simulink model "simulation"  (R2019b)
settings: Solver=VariableStepAuto  StartTime=0.0  StopTime=25.0  RelTol=1e-3
values from neighbouring files (symbols this model uses):
  beta = [b_gb_lw; b_gb_rw; b_t]    [config.m]
  g = 9.8    [config.m]
  J = [Jbphi; Jbpsi; Jm; Jw]    [config.m]
  K_enc = 1    [config.m]
  K_gyro = 1    [config.m]
  M = [Mb; Mw]    [config.m]
  params = [L; W; R; eta]    [config.m]
  Q = 10    [NMPC_controller.m]    (also in config.m = eta*K_mot*K_da*[K_amp_lw, 0; 0, K_amp_rw; -K_amp_lw, -K_amp_)
  q_dot_inital = [0; 0; 0]    [config.m]
  q_inital = [0; 0; 0]    [config.m]
undefined symbols (not defined in the file or in its folder): q_dot_initial, q_initial, sigbuilder_block, x_initial, y_initial
libraries: simulink x1
settings Model: Creator=nishantmittal  LastModifiedBy=nishantmittal

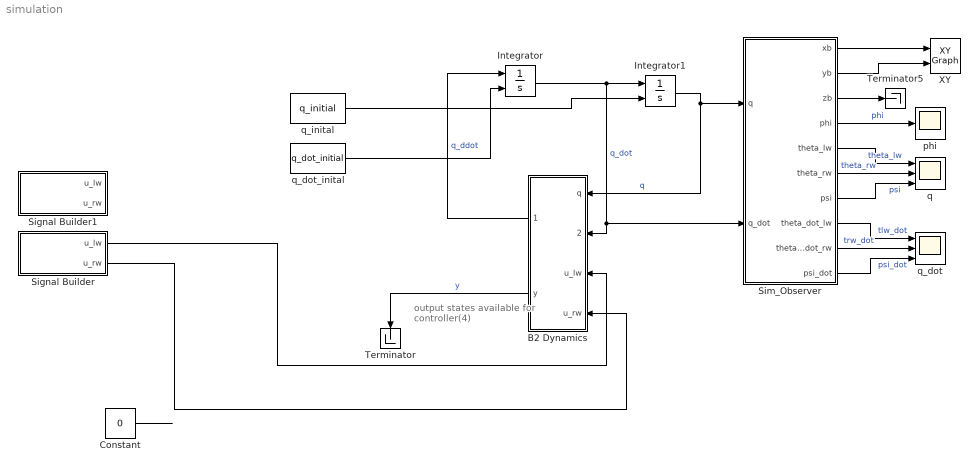
== system simulation ==
  note: output states available
      | for controller(4)
  "B2 Dynamics " : Subsystem
  Constant : Constant  Value=0
  Integrator : Integrator  InitialConditionSource=external  InitialCondition=q_dot_inital
  Integrator1 : Integrator  InitialConditionSource=external  InitialCondition=q_inital
  Signal Builder : Subsystem  Tag=STV Subsys  LoadFcn=sigbuilder_block('load');  StartFcn=sigbuilder_block('start');  StopFcn=sigbuilder_block('stop');  ClipboardFcn=sigbuilder_block('clipboard');  mask(Sigbuilder block){tuvar=[0:10]}
      mask help: Simulink:masks:SigbuilderBlock_MD
      mask init:
      | if ~strcmp(get_param(bdroot(gcbh),'SimulationStatus'),'stopped') tuvar = sigbuilder_block('maskInit'); end
      settings: CopyFcn=sigbuilder_block('copy');  DeleteFcn=sigbuilder_block('delete');  ModelCloseFcn=sigbuilder_block('modelClose');  PreSaveFcn=sigbuilder_block('preSave');  PauseFcn=sigbuilder_block('pause');  ContinueFcn=sigbuilder_block('continue');  NameChangeFcn=sigbuilder_block('namechange');  OpenFcn=sigbuilder_block('open',[436 201 612 537 ]);  CloseFcn=sigbuilder_block('close');
      mask Display: plot(0, 0, 100, 100,[2, 2, 32, 32, 2], [68, 8, 8, 68, 68],[32, 2], [38, 38], [32, 19, 2],[53, 60, 44], [32, 17, 17, 2],[16, 16, 31, 31]);txt = getActiveGroup(gcbh);text(2, 100, txt,'verticalAlignment', 'top');
  Signal Builder1 : Subsystem  Tag=STV Subsys  LoadFcn=sigbuilder_block('load');  StartFcn=sigbuilder_block('start');  StopFcn=sigbuilder_block('stop');  ClipboardFcn=sigbuilder_block('clipboard');  mask(Sigbuilder block){tuvar=[0:10]}
      mask help: Simulink:masks:SigbuilderBlock_MD
      mask init:
      | if ~strcmp(get_param(bdroot(gcbh),'SimulationStatus'),'stopped') tuvar = sigbuilder_block('maskInit'); end
      settings: CopyFcn=sigbuilder_block('copy');  DeleteFcn=sigbuilder_block('delete');  ModelCloseFcn=sigbuilder_block('modelClose');  PreSaveFcn=sigbuilder_block('preSave');  PauseFcn=sigbuilder_block('pause');  ContinueFcn=sigbuilder_block('continue');  NameChangeFcn=sigbuilder_block('namechange');  OpenFcn=sigbuilder_block('open',[436 201 612 537 ]);  CloseFcn=sigbuilder_block('close');
      mask Display: plot(0, 0, 100, 100,[2, 2, 32, 32, 2], [68, 8, 8, 68, 68],[32, 2], [38, 38], [32, 19, 2],[53, 60, 44], [32, 17, 17, 2],[16, 16, 31, 31]);txt = getActiveGroup(gcbh);text(2, 100, txt,'verticalAlignment', 'top');
  Sim_Observer : Subsystem
  Terminator : Terminator
  Terminator5 : Terminator
  XY : simulink/Sinks/XY Graph  xmin=-25  xmax=25  ymin=-25  ymax=25  st=-1
  phi : Scope
  q : Scope  NumInputPorts=3
  q_dot : Scope  NumInputPorts=3
  q_dot_inital : Constant  Value=q_dot_initial
  q_inital : Constant  Value=q_initial
  wires:
  Integrator/1 -> "B2 Dynamics "/2(q_dot), Sim_Observer/2(q_dot), Integrator1/1  "q_dot"
  Integrator1/1 -> Sim_Observer/1(q), "B2 Dynamics "/1(q)  "q"
  "B2 Dynamics "/1(q_ddot) -> Integrator/1  "q_ddot"
  "B2 Dynamics "/2(y) -> Terminator/1  "y"
  q_dot_inital/1 -> Integrator/2
  q_inital/1 -> Integrator1/2
  Sim_Observer/6(theta_rw) -> q/2  "theta_rw"
  Sim_Observer/5(theta_lw) -> q/1  "theta_lw"
  Sim_Observer/7(psi) -> q/3  "psi"
  Sim_Observer/2(yb) -> XY/2
  Sim_Observer/1(xb) -> XY/1
  Sim_Observer/10(psi_dot) -> q_dot/3  "psi_dot"
  Sim_Observer/9(theta_dot_rw) -> q_dot/2  "trw_dot"
  Sim_Observer/8(theta_dot_lw) -> q_dot/1  "tlw_dot"
  Sim_Observer/4("phi ") -> phi/1  "phi"
  Sim_Observer/3(zb) -> Terminator5/1
  Constant/1 -> ?
  Signal Builder/1(u_lw) -> "B2 Dynamics "/3(u_lw)
  Signal Builder/2(u_rw) -> "B2 Dynamics "/4(u_rw)

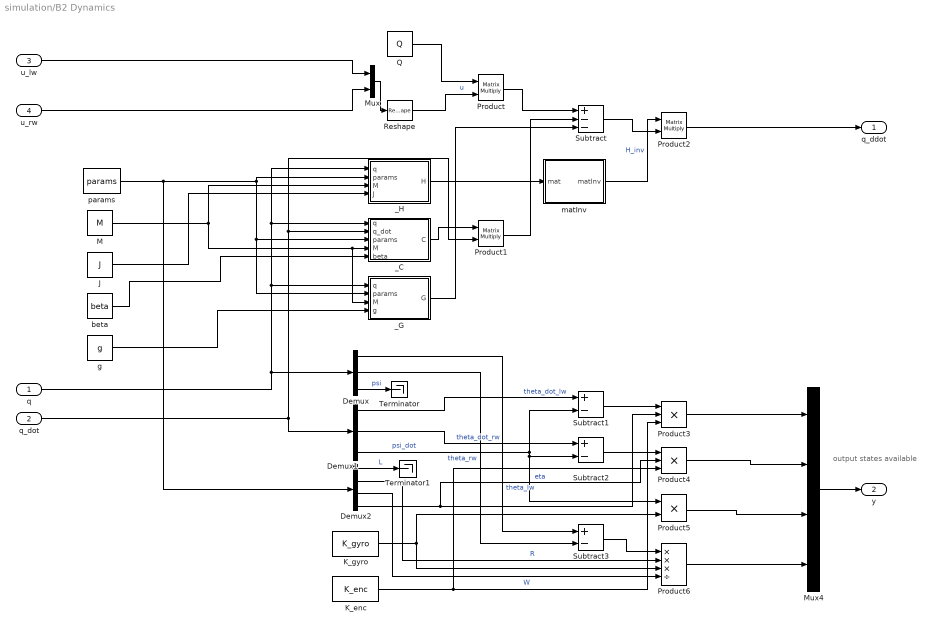
== system simulation/B2 Dynamics  ==
  note: output states available
  q : Inport
  q_dot : Inport  Port=2
  u_lw : Inport  Port=3
  u_rw : Inport  Port=4
  Demux : Demux  Outputs=3
  Demux1 : Demux  Outputs=3
  Demux2 : Demux
  J : Constant  Value=J
  K_enc : Constant  Value=K_enc
  K_gyro : Constant  Value=K_gyro
  M : Constant  Value=M
  Mux : Mux  Inputs=2
  Mux4 : Mux
  Product : Product  Multiplication=Matrix(*)
  Product1 : Product  Multiplication=Matrix(*)
  Product2 : Product  Multiplication=Matrix(*)
  Product3 : Product  Inputs=3
  Product4 : Product  Inputs=3
  Product5 : Product
  Product6 : Product  Inputs=***/
  Q : Constant  Value=Q
  Reshape : Reshape  OutputDimensionality=Column vector (2-D)
  Subtract : Sum  Inputs=+--
  Subtract1 : Sum  Inputs=+-
  Subtract2 : Sum  Inputs=+-
  Subtract3 : Sum  Inputs=+-
  Terminator : Terminator
  Terminator1 : Terminator
  _C : MATLAB Function  TreatAsAtomicUnit=on
  _G : MATLAB Function  TreatAsAtomicUnit=on
  _H : MATLAB Function  TreatAsAtomicUnit=on
  beta : Constant  Value=beta
  g : Constant  Value=g
  matInv : MATLAB Function  TreatAsAtomicUnit=on
  "params " : Constant  Value=params
  q_ddot : Outport
  y : Outport  Port=2
  wires:
  q_dot/1 -> _C/2(q_dot), Product1/2, Demux1/1
  "params "/1 -> Demux2/1, _G/2(params), _C/3(params), _H/2(params)
  beta/1 -> _C/5(beta)
  J/1 -> _H/4(J)
  M/1 -> _H/3(M), _G/3(M), _C/4(M)
  g/1 -> _G/4(g)
  u_rw/1 -> Mux/2
  u_lw/1 -> Mux/1
  Mux/1 -> Reshape/1
  _H/1(H) -> matInv/1(mat)
  Product/1 -> Subtract/1
  Product1/1 -> Subtract/2
  _G/1(G) -> Subtract/3
  Product2/1 -> q_ddot/1
  Demux/1 -> Subtract3/1  "theta_lw"
  Demux/2 -> Subtract3/2  "theta_rw"
  Demux1/1 -> Subtract1/1  "theta_dot_lw"
  Subtract1/1 -> Product3/1
  Demux2/2 -> Product6/2  "R"
  Demux2/3 -> Product6/4  "W"
  K_enc/1 -> Product4/3, Product3/3
  Demux1/2 -> Subtract2/1  "theta_dot_rw"
  Subtract2/1 -> Product4/1
  Demux2/4 -> Product4/2, Product3/2  "eta"
  Demux1/3 -> Subtract1/2, Product5/1, Subtract2/2  "psi_dot"
  K_gyro/1 -> Product5/2, Product6/3
  Subtract3/1 -> Product6/1
  Product3/1 -> Mux4/1
  Product4/1 -> Mux4/2
  Product5/1 -> Mux4/3
  Product6/1 -> Mux4/4
  Mux4/1 -> y/1
  Reshape/1 -> Product/2  "u"
  Q/1 -> Product/1
  Subtract/1 -> Product2/2
  matInv/1(matInv) -> Product2/1  "H_inv"
  _C/1(C) -> Product1/1
  Demux/3 -> Terminator/1  "psi"
  Demux2/1 -> Terminator1/1  "L"
  q/1 -> _H/1(q), _C/1(q), _G/1(q), Demux/1

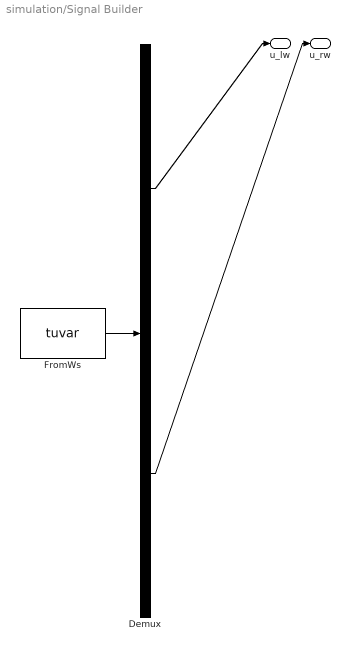
== system simulation/Signal Builder ==
  Demux : Demux  Tag=STV Demux  Outputs=2
  FromWs : FromWorkspace  Tag=STV FromWs  VariableName=tuvar  SampleTime=0
      SigBuilderData=|
      | common.afterFinalStr = 'Extrapolate'
      | common.sampleTime = 0
      | dataSet.timeRange = [0 10]
      | dataSet.name = 'Rotaate'
      | sbobj.Groups.Name = 'Rotaate'
      | sbobj.Groups.Signals(1).Name = 'u_lw'
      | sbobj.Groups.Signals(1).XData = [0 1 1 2 2 3 3 10]
      | sbobj.Groups.Signals(1).YData = [0 0 1.56 1.56 -1.54 -1.54 0 0]
      | sbobj.Groups.Signals(2).Name = 'u_rw'
      | sbobj.Groups.Signals(2).XData = [0 1 1 2 2 3 3 10]
      | sbobj.Groups.Signals(2).YData = [0 0 -1.56 -1.56 1.56 1.56 0 0]
  u_lw : Outport  Tag=STV Outport
  u_rw : Outport  Tag=STV Outport  Port=2
  wires:
  FromWs/1 -> Demux/1
  Demux/1 -> u_lw/1
  Demux/2 -> u_rw/1

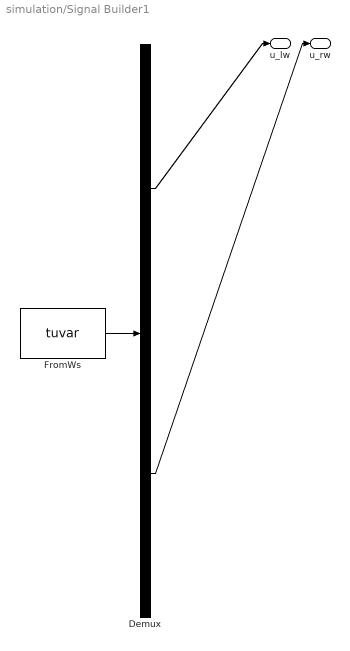
== system simulation/Signal Builder1 ==
  Demux : Demux  Tag=STV Demux  Outputs=2
  FromWs : FromWorkspace  Tag=STV FromWs  VariableName=tuvar  SampleTime=0
      SigBuilderData=|
      | common.afterFinalStr = 'Extrapolate'
      | common.sampleTime = 0
      | dataSet(1).timeRange = [0 10]
      | dataSet(1).name = 'Forward_back'
      | dataSet(2).timeRange = [0 10]
      | dataSet(2).name = 'Group 2'
      | sbobj.Groups(1).Name = 'Forward_back'
      | sbobj.Groups(1).Signals(1).Name = 'u_lw'
      | sbobj.Groups(1).Signals(1).XData = [0 1 1 2 2 3 3 10]
      | sbobj.Groups(1).Signals(1).YData = [0 0 1.56 1.56 -1.54 -1.54 0 0]
      | sbobj.Groups(1).Signals(2).Name = 'u_rw'
      | sbobj.Groups(1).Signals(2).XData = [0 1 1 2 2 3 3 10]
      | sbobj.Groups(1).Signals(2).YData = [0 0 1.56 1.56 -1.56 -1.56 0 0]
      | sbobj.Groups(2).Name = 'Group 2'
      | sbobj.Groups(2).Signals(1).Name = 'u_lw'
      | sbobj.Groups(2).Signals(1).XData = [0 1 1 2 2 3 3 10]
      | sbobj.Groups(2).Signals(1).YData = [0 0 1 1 -1 -1 0 0]
      | sbobj.Groups(2).Signals(2).Name = 'u_rw'
      | sbobj.Groups(2).Signals(2).XData = [0 1 1 2 2 3 3 10]
      | sbobj.Groups(2).Signals(2).YData = [0 0 1 1 -1 -1 0 0]
  u_lw : Outport  Tag=STV Outport
  u_rw : Outport  Tag=STV Outport  Port=2
  wires:
  FromWs/1 -> Demux/1
  Demux/1 -> u_lw/1
  Demux/2 -> u_rw/1

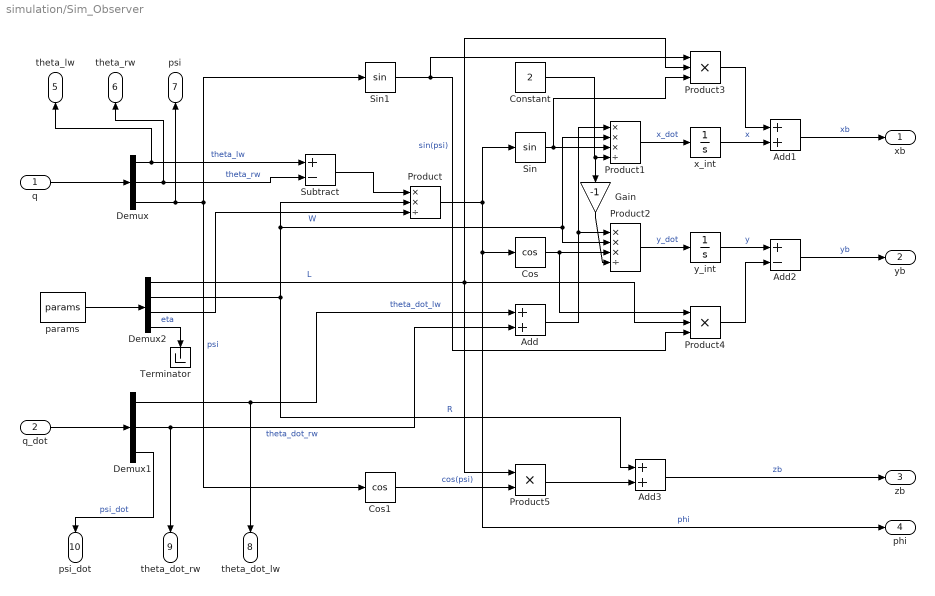
== system simulation/Sim_Observer ==
  q : Inport
  q_dot : Inport  Port=2
  Add : Sum
  Add1 : Sum
  Add2 : Sum  Inputs=+-
  Add3 : Sum
  Constant : Constant  Value=2
  Cos : Trigonometry  Operator=cos
  Cos1 : Trigonometry  Operator=cos
  Demux : Demux  Outputs=3
  Demux1 : Demux  Outputs=3
  Demux2 : Demux
  Gain : Gain  Gain=-1
  Product : Product  Inputs=**/
  Product1 : Product  Inputs=***/
  Product2 : Product  Inputs=***/
  Product3 : Product  Inputs=3
  Product4 : Product  Inputs=3
  Product5 : Product
  Sin : Trigonometry
  Sin1 : Trigonometry
  Subtract : Sum  Inputs=+-
  Terminator : Terminator
  "params " : Constant  Value=params
  x_int : Integrator  InitialCondition=x_initial
  y_int : Integrator  InitialCondition=y_initial
  xb : Outport
  yb : Outport  Port=2
  zb : Outport  Port=3
  "phi " : Outport  Port=4
  theta_lw : Outport  Port=5
  theta_rw : Outport  Port=6
  psi : Outport  Port=7
  theta_dot_lw : Outport  Port=8
  theta_dot_rw : Outport  Port=9
  psi_dot : Outport  Port=10
  wires:
  q/1 -> Demux/1
  Demux/1 -> theta_lw/1, Subtract/1  "theta_lw"
  Demux/2 -> Subtract/2, theta_rw/1  "theta_rw"
  Demux/3 -> Sin1/1, Cos1/1, psi/1  "psi"
  q_dot/1 -> Demux1/1
  Demux1/1 -> theta_dot_lw/1, Add/1  "theta_dot_lw"
  Demux1/2 -> Add/2, theta_dot_rw/1  "theta_dot_rw"
  Demux1/3 -> psi_dot/1  "psi_dot"
  "params "/1 -> Demux2/1
  Demux2/1 -> Product5/1, Product4/2, Product3/2  "L"
  Demux2/2 -> Add3/1, Product2/2, Product1/2, Product/2  "R"
  Demux2/3 -> Product/3  "W"
  Demux2/4 -> Terminator/1  "eta"
  Subtract/1 -> Product/1
  Product/1 -> "phi "/1, Cos/1, Sin/1  "phi"
  Sin/1 -> Product3/3, Product1/3
  Cos/1 -> Product4/1, Product2/3
  Add/1 -> Product2/1, Product1/1
  Constant/1 -> Gain/1, Product1/4
  Gain/1 -> Product2/4
  Product1/1 -> x_int/1  "x_dot"
  Product2/1 -> y_int/1  "y_dot"
  Sin1/1 -> Product4/3, Product3/1  "sin(psi)"
  y_int/1 -> Add2/1  "y"
  Product4/1 -> Add2/2
  x_int/1 -> Add1/2  "x"
  Product3/1 -> Add1/1
  Cos1/1 -> Product5/2  "cos(psi)"
  Add1/1 -> xb/1  "xb"
  Add2/1 -> yb/1  "yb"
  Product5/1 -> Add3/2
  Add3/1 -> zb/1  "zb"

== matlab function simulation/B2 Dynamics /_G ==
  data: q input; params input; M input; G output; g input
function G = fcn(q, params, M, g)

%Returns G(q)
% q contains the current state
% params are the parmeters params = [L, W, R, eta]
% M is the mass vector M = [Mb, Mw,]
% g is acceleration due to gravity

tlw = q(1);
trw = q(2);
psi = q(3);

L = params(1);
W = params(2);
R = params(3);
eta = params(4);

Mb = M(1);
Mw = M(2);

G = [0; 0; -g*L*Mb*sin(psi)];

== matlab function simulation/B2 Dynamics /_C ==
  data: q input; C output; q_dot input; params input; M input; beta input
function C = fcn(q, q_dot, params, M, beta)

%Returns C(q, \dot q) 
% q contains the current state
% q_dot contains the current state rate
% params are the parmeters params = [L, W, R, eta]
% M is the mass vector M = [Mb, Mw,]
% beta contains friction info beta = [b_gb_stiction; b_gb_coloumb; b_gb_viscous; b_t];

tlw = q(1);
trw = q(2);
psi = q(3);

tlw_dot = q_dot(1);
trw_dot = q_dot(2);
psi_dot = q_dot(3);

L = params(1);
W = params(2);
R = params(3);
eta = params(4);

Mb = M(1);
Mw = M(2);

b_gb_stiction = beta(1);
b_gb_coloumb = beta(2);
b_gb_viscous = beta(3);
b_t = beta(4);

ca = L^2*R^2*Mb*sin(2*psi)*psi_dot/W^2;
cb = -W^2*sec(psi)/(4*L*R);
if psi_dot ~= 0
    cc = (tlw_dot - trw_dot)/(2*psi_dot);
else
    cc = 0;
end

if tlw_dot == 0
    b_gblw = b_gb_stiction;
elseif tlw_dot > 0
    b_gblw = b_gb_coloumb + b_gb_viscous*tlw_dot;
else
    b_gblw = -b_gb_coloumb + b_gb_viscous*tlw_dot;
end

if trw_dot == 0
    b_gbrw = b_gb_stiction;
elseif trw_dot > 0
    b_gbrw = b_gb_coloumb + b_gb_viscous*tlw_dot;
else
    b_gbrw = -b_gb_coloumb + b_gb_viscous*tlw_dot;
end
     

C = ca*[1, -1, cb; -1, 1, cb; -cc, cc, 0] + [(b_gblw + b_t), 0, (-b_gblw); 0, (b_gbrw + b_t), (-b_gbrw); (-b_gblw), (-b_gbrw), (b_gblw + b_gbrw)];

== matlab function simulation/B2 Dynamics /_H ==
  data: q input; params input; M input; H output; J input
function H = fcn(q, params, M, J)

%Returns H(q) 
%   q contains the current state
% params are the parmeters params = [L, W, R, eta]
% M is the mass vector M = [Mb, Mw,]
% J is the intertia vector J = [Jbphi, Jbpsi, Jm, Jw]

tlw = q(1);
trw = q(2);
psi = q(3);

L = params(1);
W = params(2);
R = params(3);
eta = params(4);

Mb = M(1);
Mw = M(2);

Jbphi = J(1);
Jbpsi = J(2);
Jm = J(3);
Jw = J(4);

ha = 1/(4*W^2);
hb = L*R*Mb*cos(psi)/(2);
hc = L^2*R^2*Mb*cos(2*psi)/(2*W^2);

h0 = (4*Mw*W^2 + 4*Jbphi + (2*L^2 + W^2)*Mb)*R^2 + 4*W^2*(Jm*eta^2 +Jw);
h1 = (Mb*(W^2 - 2*L^2) - 4*Jbphi)*R^2;
h2 = -4*W^2*eta^2*Jm;
h3 = 4*W^2*(Mb*L^2 + Jbpsi + 2*eta^2*Jm);

H = ha*[h0, h1, h2; h1, h0, h2; h2, h2, h3] + [-ha, hc, hb; hc, -hc, hb; hb, hb 0];

== matlab function simulation/B2 Dynamics /matInv ==
  data: mat input; matInv output
function matInv = fcn(mat)

%Returns inverse of the matrix
% if inv does not exist - throws warning

matInv = inv(mat);
